simulink library "Nav_sys"  (R2018b)
settings: Solver=VariableStepAuto  StartTime=0.0  StopTime=10.0  RelTol=1e-3
values from neighbouring files (symbols this model uses):
  Lookah_distance = 40    [big_pam.m]
  Waypont = [ 0	0	hightz	0	; 20	0	hightz	0	; 20	5	hightz	0	; 0	5	hightz	0	; 0	10	hightz	0	; 20	10	hightz	0	; 20	15	hightz	0	; 0	15	hightz	0	; 0	20	hightz	0	; 20	20	hightz	0	; 20	25	hightz	0	; 0	25	hightz	0	]    [big_pam.m]
libraries: simulink x2, robotuavlib x1
settings Model: Creator=Andrew Garcia  LastModifiedBy=Andrew Garcia

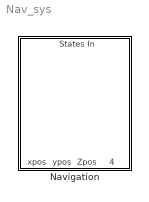
== system Nav_sys ==
  Navigation : Subsystem  LoadFcn=big_pam  InitFcn=big_pam

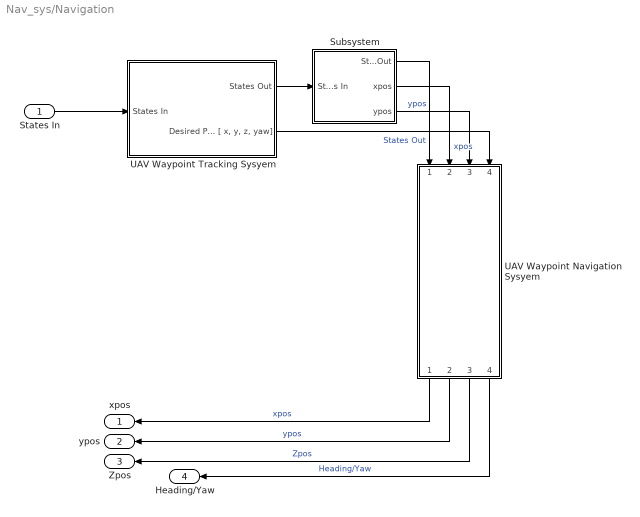
== system Nav_sys/Navigation ==
  States In : Inport
  Subsystem : Subsystem
  "UAV Waypoint Navigation Sysyem " : Subsystem
  "UAV Waypoint Tracking Sysyem " : Subsystem
  xpos : Outport
  ypos : Outport  Port=2
  Zpos : Outport  Port=3
  Heading/Yaw : Outport  Port=4
  wires:
  States In/1 -> "UAV Waypoint Tracking Sysyem "/1(States In)
  "UAV Waypoint Navigation Sysyem "/1(Xpos) -> xpos/1  "xpos"
  "UAV Waypoint Tracking Sysyem "/1(States Out) -> Subsystem/1(States In)
  "UAV Waypoint Navigation Sysyem "/2(Ypos) -> ypos/1  "ypos"
  Subsystem/1(States* Out) -> "UAV Waypoint Navigation Sysyem "/1(States* In)  "States Out"
  "UAV Waypoint Tracking Sysyem "/2("Desired Position [ x, y, z, yaw]") -> "UAV Waypoint Navigation Sysyem "/4("Desired Pos In [ x, y, z, yaw]")
  Subsystem/3(ypos) -> "UAV Waypoint Navigation Sysyem "/3(ypos)  "ypos"
  Subsystem/2(xpos) -> "UAV Waypoint Navigation Sysyem "/2(xpos)  "xpos"
  "UAV Waypoint Navigation Sysyem "/3(Zpos) -> Zpos/1  "Zpos"
  "UAV Waypoint Navigation Sysyem "/4(Heading/Yaw [Rad]) -> Heading/Yaw/1  "Heading/Yaw"

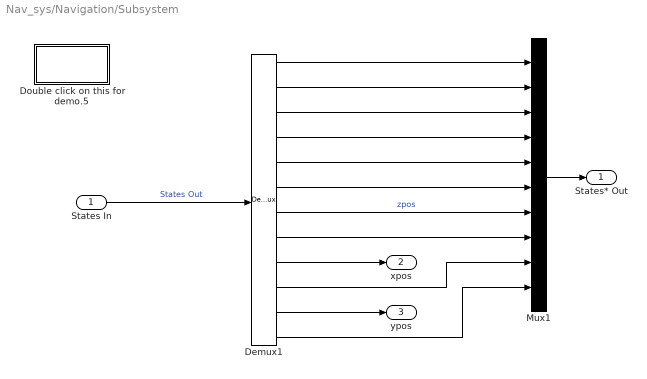
== system Nav_sys/Navigation/Subsystem ==
  States In : Inport
  Demux1 : Demux  Outputs=12
  Double click on this for demo.5 : Subsystem
      settings: OpenFcn=optsiminit
      mask Display: disp('optsiminit')
  Mux1 : Mux  Inputs=10
  States* Out : Outport
  xpos : Outport  Port=2
  ypos : Outport  Port=3
  wires:
  States In/1 -> Demux1/1  "States Out"
  Demux1/11 -> ypos/1
  Demux1/9 -> xpos/1
  Mux1/1 -> States* Out/1
  Demux1/12 -> Mux1/10
  Demux1/10 -> Mux1/9
  Demux1/8 -> Mux1/8
  Demux1/7 -> Mux1/7  "zpos"
  Demux1/6 -> Mux1/6
  Demux1/5 -> Mux1/5
  Demux1/4 -> Mux1/4
  Demux1/3 -> Mux1/3
  Demux1/2 -> Mux1/2
  Demux1/1 -> Mux1/1

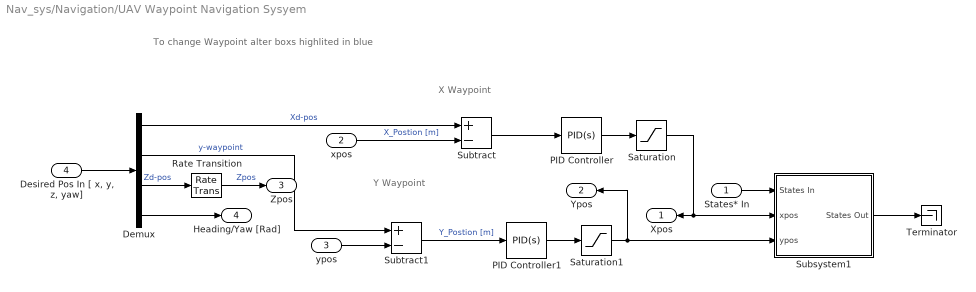
== system Nav_sys/Navigation/UAV Waypoint Navigation Sysyem  ==
  note: X Waypoint
  note: Y Waypoint
  note: To change Waypoint alter boxs highlited in blue
  States* In : Inport
  xpos : Inport  Port=2
  ypos : Inport  Port=3
  "Desired Pos In [ x, y, z, yaw]" : Inport  Port=4
  Demux : Demux
  PID Controller : simulink/Continuous/PID Controller  Controller=PID  Form=Parallel  TimeDomain=Continuous-time  SampleTime=-1  IntegratorMethod=Forward Euler  FilterMethod=Forward Euler  ControllerParametersSource=internal  P=0.8  I=0.2  D=0  UseFilter=on  N=100  TunerSelectOption=Transfer Function Based (PID Tuner App)  InitialConditionSource=internal  InitialConditionForIntegrator=0  InitialConditionForFilter=0  DifferentiatorICPrevScaledInput=0  ExternalReset=none  TrackingMode=off  Kt=1  LimitOutput=off  UpperSaturationLimit=inf  LowerSaturationLimit=-inf  LinearizeAsGain=off  AntiWindupMode=none  Kb=1  POutMin=[]  POutMax=[]  IOutMin=[]  IOutMax=[]  DOutMin=[]  DOutMax=[]  NOutMin=[]  NOutMax=[]  SumOutMin=[]  SumOutMax=[]  SaturationOutMin=[]  SaturationOutMax=[]  PParamMin=[]  PParamMax=[]  IParamMin=[]  IParamMax=[]  DParamMin=[]  DParamMax=[]  NParamMin=[]  NParamMax=[]  KbParamMin=[]  KbParamMax=[]  KtParamMin=[]  KtParamMax=[]  KbOutMin=[]  KbOutMax=[]  KtOutMin=[]  KtOutMax=[]  IntegratorOutMin=[]  IntegratorOutMax=[]  FilterOutMin=[]  FilterOutMax=[]  SumI1OutMin=[]  SumI1OutMax=[]  SumI2OutMin=[]  SumI2OutMax=[]  SumI3OutMin=[]  SumI3OutMax=[]  SumI4OutMin=[]  SumI4OutMax=[]  SumDOutMin=[]  SumDOutMax=[]  DifferentiatorOutMin=[]  DifferentiatorOutMax=[]  FilterDiffOutCoefMin=[]  FilterDiffOutCoefMax=[]  ReciprocalOutMin=[]  ReciprocalOutMax=[]  SumDenOutMin=[]  SumDenOutMax=[]  SumNumOutMin=[]  SumNumOutMax=[]  DivideOutMin=[]  DivideOutMax=[]  IntegratorContinuousStateAttributes=''  IntegratorStateMustResolveToSignalObject=off  IntegratorRTWStateStorageClass=Auto  FilterContinuousStateAttributes=''  FilterStateMustResolveToSignalObject=off  FilterRTWStateStorageClass=Auto  ParallelPVariant=InternalParameters  IdealPVariant=Disabled  IVariant=InternalParameters  DVariant=InternalParameters  IntegratorVariant=Continuous  SatVariant=Disabled  AWVariant=Passthrough  PCopyVariant=Disabled  TRVariant=Disabled  FdbkBlocksVariant=Forward  IdealPFdbkVariant=Disabled  SatFdbkVariant=Disabled  DerivativeFilterVariant=ContFilter  NVariant=InternalParameters  NCopyVariant=Disabled  FilterICVariant=InternalICsFilter  IntegratorICVariant=InternalICs  ExternalResetVariant=Disabled  TRSumVariant=Passthrough  SumFdbkVariant=Disabled  SumVariant=Sum_PID
  PID Controller1 : simulink/Continuous/PID Controller  Controller=PID  Form=Parallel  TimeDomain=Continuous-time  SampleTime=-1  IntegratorMethod=Forward Euler  FilterMethod=Forward Euler  ControllerParametersSource=internal  P=1  I=0.2  D=0  UseFilter=on  N=100  TunerSelectOption=Transfer Function Based (PID Tuner App)  InitialConditionSource=internal  InitialConditionForIntegrator=0  InitialConditionForFilter=0  DifferentiatorICPrevScaledInput=0  ExternalReset=none  TrackingMode=off  Kt=1  LimitOutput=off  UpperSaturationLimit=inf  LowerSaturationLimit=-inf  LinearizeAsGain=off  AntiWindupMode=none  Kb=1  POutMin=[]  POutMax=[]  IOutMin=[]  IOutMax=[]  DOutMin=[]  DOutMax=[]  NOutMin=[]  NOutMax=[]  SumOutMin=[]  SumOutMax=[]  SaturationOutMin=[]  SaturationOutMax=[]  PParamMin=[]  PParamMax=[]  IParamMin=[]  IParamMax=[]  DParamMin=[]  DParamMax=[]  NParamMin=[]  NParamMax=[]  KbParamMin=[]  KbParamMax=[]  KtParamMin=[]  KtParamMax=[]  KbOutMin=[]  KbOutMax=[]  KtOutMin=[]  KtOutMax=[]  IntegratorOutMin=[]  IntegratorOutMax=[]  FilterOutMin=[]  FilterOutMax=[]  SumI1OutMin=[]  SumI1OutMax=[]  SumI2OutMin=[]  SumI2OutMax=[]  SumI3OutMin=[]  SumI3OutMax=[]  SumI4OutMin=[]  SumI4OutMax=[]  SumDOutMin=[]  SumDOutMax=[]  DifferentiatorOutMin=[]  DifferentiatorOutMax=[]  FilterDiffOutCoefMin=[]  FilterDiffOutCoefMax=[]  ReciprocalOutMin=[]  ReciprocalOutMax=[]  SumDenOutMin=[]  SumDenOutMax=[]  SumNumOutMin=[]  SumNumOutMax=[]  DivideOutMin=[]  DivideOutMax=[]  IntegratorContinuousStateAttributes=''  IntegratorStateMustResolveToSignalObject=off  IntegratorRTWStateStorageClass=Auto  FilterContinuousStateAttributes=''  FilterStateMustResolveToSignalObject=off  FilterRTWStateStorageClass=Auto  ParallelPVariant=InternalParameters  IdealPVariant=Disabled  IVariant=InternalParameters  DVariant=InternalParameters  IntegratorVariant=Continuous  SatVariant=Disabled  AWVariant=Passthrough  PCopyVariant=Disabled  TRVariant=Disabled  FdbkBlocksVariant=Forward  IdealPFdbkVariant=Disabled  SatFdbkVariant=Disabled  DerivativeFilterVariant=ContFilter  NVariant=InternalParameters  NCopyVariant=Disabled  FilterICVariant=InternalICsFilter  IntegratorICVariant=InternalICs  ExternalResetVariant=Disabled  TRSumVariant=Passthrough  SumFdbkVariant=Disabled  SumVariant=Sum_PID
  Rate Transition : RateTransition
  Saturation : Saturate  UpperLimit=20  LowerLimit=-20
  Saturation1 : Saturate  UpperLimit=20  LowerLimit=-20
  Subsystem1 : Subsystem
  Subtract : Sum  Inputs=+-
  Subtract1 : Sum  Inputs=+-
  Terminator : Terminator
  Xpos : Outport
  Ypos : Outport  Port=2
  Zpos : Outport  Port=3
  Heading/Yaw [Rad] : Outport  Port=4
  wires:
  Demux/3 -> Rate Transition/1  "Zd-pos"
  Demux/1 -> Subtract/1  "Xd-pos"
  "Desired Pos In [ x, y, z, yaw]"/1 -> Demux/1
  ypos/1 -> Subtract1/2
  Rate Transition/1 -> Zpos/1  "Zpos"
  States* In/1 -> Subsystem1/1(States In)
  xpos/1 -> Subtract/2  "X_Postion [m]"
  Demux/4 -> Heading/Yaw [Rad]/1
  PID Controller/1 -> Saturation/1
  Saturation1/1 -> Ypos/1, Subsystem1/3(ypos)
  Demux/2 -> Subtract1/1  "y-waypoint"
  PID Controller1/1 -> Saturation1/1
  Subsystem1/1(States Out) -> Terminator/1
  Subtract/1 -> PID Controller/1
  Subtract1/1 -> PID Controller1/1  "Y_Postion [m]"
  Saturation/1 -> Xpos/1, Subsystem1/2(xpos)

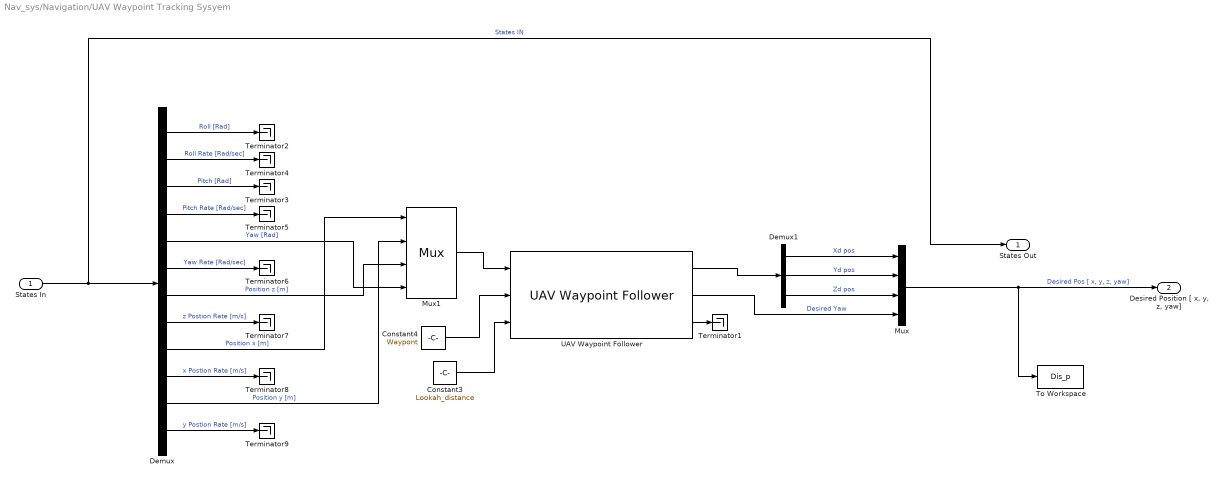
== system Nav_sys/Navigation/UAV Waypoint Tracking Sysyem  ==
  States In : Inport
  Constant3 : Constant  Value=Lookah_distance
  Constant4 : Constant  Value=Waypont
  Demux : Demux  Outputs=12
  Demux1 : Demux  Outputs=3
  Mux : Mux
  Mux1 : Mux
      settings: DisplayOption=signals
  Terminator{1..9} (9 alike) : Terminator
  To Workspace : ToWorkspace  VariableName=Dis_p  SaveFormat=Timeseries  SampleTime=-1
  UAV Waypoint Follower : robotuavlib/UAV Waypoint Follower  UAVType=multirotor  StartFrom=closest  TransitionRadiusSource=internal  TransitionRadius=5  YawInput=on  ShowCrossTrackErrorOutput=off  ShowStatusOutput=off  SimulateUsing=Interpreted execution
      settings: SourceProductName=Robotics System Toolbox UAV Library
  States Out : Outport
  "Desired Position [ x, y, z, yaw]" : Outport  Port=2
  wires:
  Mux1/1 -> UAV Waypoint Follower/1
  Mux/1 -> To Workspace/1, "Desired Position [ x, y, z, yaw]"/1  "Desired Pos [ x, y, z, yaw]"
  UAV Waypoint Follower/3 -> Terminator1/1
  Demux1/3 -> Mux/3  "Zd pos"
  Demux1/1 -> Mux/1  "Xd pos"
  Constant4/1 -> UAV Waypoint Follower/2
  Constant3/1 -> UAV Waypoint Follower/3
  Demux1/2 -> Mux/2  "Yd pos"
  UAV Waypoint Follower/1 -> Demux1/1
  UAV Waypoint Follower/2 -> Mux/4  "Desired Yaw"
  Demux/7 -> Mux1/3  "Position z [m]"
  Demux/2 -> Terminator4/1  "Roll Rate [Rad/sec]"
  States In/1 -> States Out/1, Demux/1  "States IN"
  Demux/5 -> Mux1/4  "Yaw [Rad]"
  Demux/6 -> Terminator6/1  "Yaw Rate [Rad/sec]"
  Demux/10 -> Terminator8/1  "x Postion Rate [m/s]"
  Demux/3 -> Terminator3/1  "Pitch [Rad]"
  Demux/8 -> Terminator7/1  "z Postion Rate [m/s]"
  Demux/4 -> Terminator5/1  "Pitch Rate [Rad/sec]"
  Demux/9 -> Mux1/1  "Position x [m]"
  Demux/12 -> Terminator9/1  "y Postion Rate [m/s]"
  Demux/1 -> Terminator2/1  "Roll [Rad]"
  Demux/11 -> Mux1/2  "Position y [m]"

== system Nav_sys/Navigation/Subsystem/Double click on this for demo.5 ==

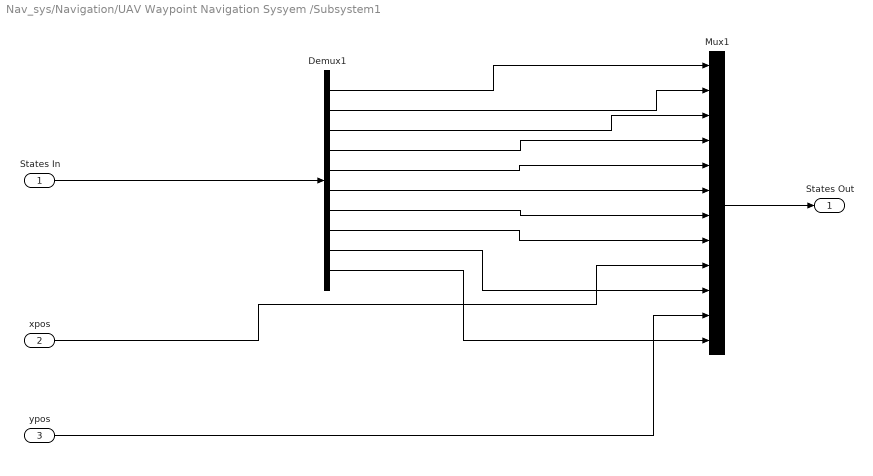
== system Nav_sys/Navigation/UAV Waypoint Navigation Sysyem /Subsystem1 ==
  States In : Inport
  xpos : Inport  Port=2
  ypos : Inport  Port=3
  Demux1 : Demux  Outputs=10
  Mux1 : Mux  Inputs=12
  States Out : Outport
  wires:
  Mux1/1 -> States Out/1
  ypos/1 -> Mux1/11
  xpos/1 -> Mux1/9
  Demux1/9 -> Mux1/10
  Demux1/10 -> Mux1/12
  Demux1/8 -> Mux1/8
  Demux1/7 -> Mux1/7
  Demux1/6 -> Mux1/6
  Demux1/5 -> Mux1/5
  Demux1/4 -> Mux1/4
  Demux1/3 -> Mux1/3
  Demux1/2 -> Mux1/2
  Demux1/1 -> Mux1/1
  States In/1 -> Demux1/1
